simulink model "Hinf_sim"  (R2020a)
settings: Solver=VariableStepAuto  StartTime=0.0  StopTime=T  MaxStep=dtmax  RelTol=1e-3
values from neighbouring files (symbols this model uses):
  b = b*b_error_scale    (= 131.4)    [Hinf_run.m]    (also in adaptive_control_run.m; passivity_fmod_run.m; passivity_velmod_run.m)
  C1 = balreal(K(1,2))    [Hinf_run.m]
  C2 = balreal(-inv(C1)*K(1,1))    [Hinf_run.m]
  input_type = 3    [Hinf_run.m]    (also in adaptive_control_run.m; passivity_fmod_run.m; passivity_velmod_run.m)
  k = k*k_error_scale    (= 11691)    [Hinf_run.m]    (also in adaptive_control_run.m; passivity_fmod_run.m; passivity_velmod_run.m)
  m = 500    [Hinf_run.m]    (also in adaptive_control_run.m; passivity_fmod_run.m; passivity_velmod_run.m)
  rampslope = 0.1    [Hinf_run.m]    (also in adaptive_control_run.m; passivity_fmod_run.m; passivity_velmod_run.m)
  sineamp = 0.1    [Hinf_run.m]    (also in adaptive_control_run.m; passivity_fmod_run.m; passivity_velmod_run.m)
  sinefreq = pi/2    (= 1.57079632679)    [Hinf_run.m]    (also in adaptive_control_run.m; passivity_fmod_run.m; passivity_velmod_run.m)
  taum = taum*taum_error_scale    (= 0.108)    [Hinf_run.m]    (also in adaptive_control_run.m; passivity_fmod_run.m; passivity_velmod_run.m)
settings Model: Creator=davidcarabis  LastModifiedBy=davidcarabis
settings DataIOCC: ReturnWorkspaceOutputs=off
settings DebuggingCC: ArithmeticOperatorsInVariantConditions=warning
settings SFSimCC: CustomCodeUndefinedFunction=UseInterfaceOnly

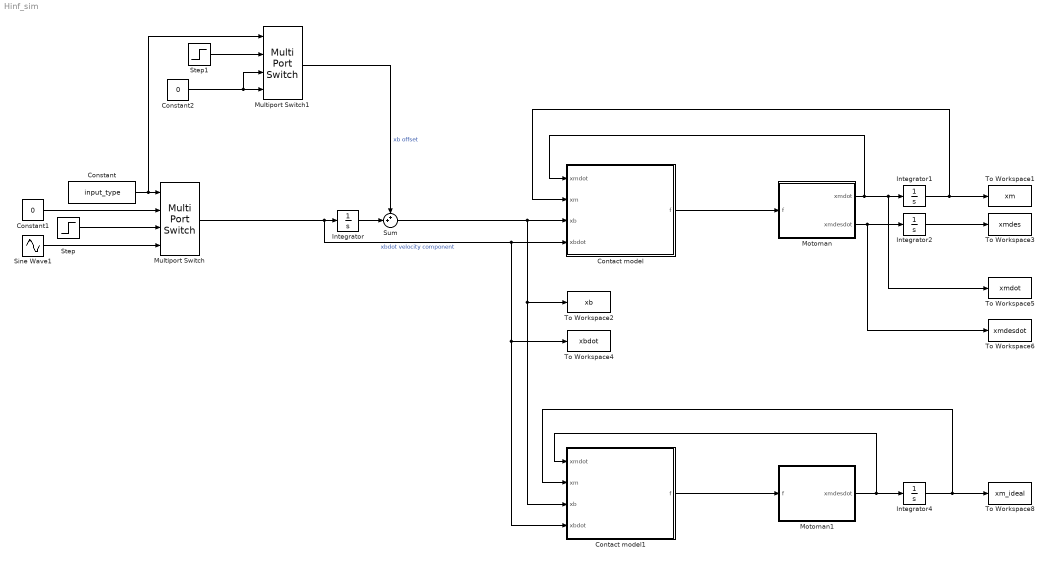
== system Hinf_sim ==
  Constant : Constant  Value=input_type
  Constant1 : Constant  Value=0
  Constant2 : Constant  Value=0
  Contact model : Subsystem
  Contact model1 : Subsystem
  Integrator{,1..2,4} (4 alike) : Integrator
  Motoman : Subsystem
  Motoman1 : Subsystem
  Multiport Switch : MultiPortSwitch
  Multiport Switch1 : MultiPortSwitch
  Sine Wave1 : Sin  Amplitude=sineamp*sinefreq  Frequency=sinefreq  Phase=pi/2  SampleTime=0
  Step : Step  Time=0  After=rampslope  SampleTime=0
  Step1 : Step  Time=0  After=rampslope  SampleTime=0
  Sum : Sum  Inputs=++|
  To Workspace1 : ToWorkspace  VariableName=xm  SampleTime=-1
  To Workspace2 : ToWorkspace  VariableName=xb
  To Workspace3 : ToWorkspace  VariableName=xmdes  SampleTime=-1
  To Workspace4 : ToWorkspace  VariableName=xbdot
  To Workspace5 : ToWorkspace  VariableName=xmdot  SampleTime=-1
  To Workspace6 : ToWorkspace  VariableName=xmdesdot  SampleTime=-1
  To Workspace8 : ToWorkspace  VariableName=xm_ideal  SampleTime=-1
  wires:
  Multiport Switch/1 -> Contact model1/4(xbdot), To Workspace4/1, Contact model/4(xbdot), Integrator/1  "xbdot velocity component"
  Constant/1 -> Multiport Switch1/1, Multiport Switch/1
  Step/1 -> Multiport Switch/3
  Sine Wave1/1 -> Multiport Switch/4
  Constant1/1 -> Multiport Switch/2
  Multiport Switch1/1 -> Sum/1  "xb offset"
  Integrator/1 -> Sum/2
  Constant2/1 -> Multiport Switch1/3, Multiport Switch1/4
  Step1/1 -> Multiport Switch1/2
  Motoman/1(xmdot) -> To Workspace5/1, Integrator1/1, Contact model/1(xmdot)
  Integrator1/1 -> Contact model/2(xm), To Workspace1/1
  Integrator2/1 -> To Workspace3/1
  Contact model/1(f) -> Motoman/1(f)
  Motoman/2(xmdesdot) -> To Workspace6/1, Integrator2/1
  Integrator4/1 -> Contact model1/2(xm), To Workspace8/1
  Contact model1/1(f) -> Motoman1/1(f)
  Motoman1/1(xmdesdot) -> Contact model1/1(xmdot), Integrator4/1
  Sum/1 -> Contact model1/3(xb), To Workspace2/1, Contact model/3(xb)

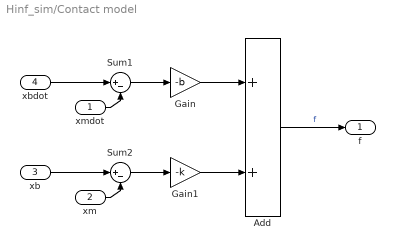
== system Hinf_sim/Contact model ==
  xmdot : Inport
  xm : Inport  Port=2
  xb : Inport  Port=3
  xbdot : Inport  Port=4
  Add : Sum
  Gain : Gain  Gain=-b
  Gain1 : Gain  Gain=-k
  Sum1 : Sum  Inputs=|+-
  Sum2 : Sum  Inputs=|+-
  f : Outport  VectorParamsAs1DForOutWhenUnconnected=off
  wires:
  xmdot/1 -> Sum1/2
  Add/1 -> f/1  "f"
  Sum2/1 -> Gain1/1
  xb/1 -> Sum2/1
  Gain1/1 -> Add/2
  Sum1/1 -> Gain/1
  xbdot/1 -> Sum1/1
  Gain/1 -> Add/1
  xm/1 -> Sum2/2

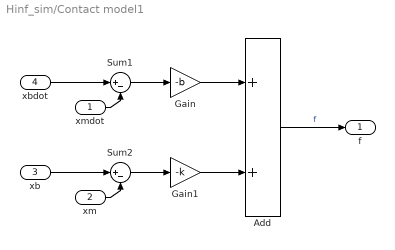
== system Hinf_sim/Contact model1 ==
  xmdot : Inport
  xm : Inport  Port=2
  xb : Inport  Port=3
  xbdot : Inport  Port=4
  Add : Sum
  Gain : Gain  Gain=-b
  Gain1 : Gain  Gain=-k
  Sum1 : Sum  Inputs=|+-
  Sum2 : Sum  Inputs=|+-
  f : Outport  VectorParamsAs1DForOutWhenUnconnected=off
  wires:
  xmdot/1 -> Sum1/2
  Add/1 -> f/1  "f"
  Sum2/1 -> Gain1/1
  xb/1 -> Sum2/1
  Gain1/1 -> Add/2
  Sum1/1 -> Gain/1
  xbdot/1 -> Sum1/1
  Gain/1 -> Add/1
  xm/1 -> Sum2/2

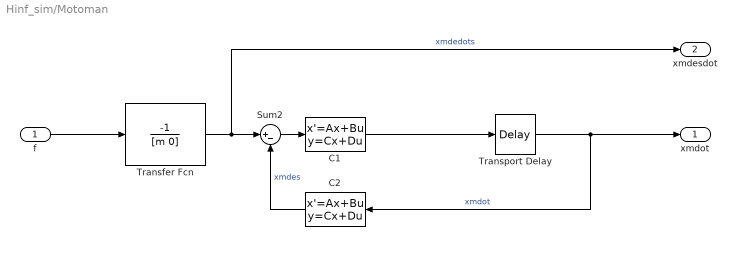
== system Hinf_sim/Motoman ==
  f : Inport
  C1 : StateSpace  A=C1.A  B=C1.B  C=C1.C  D=C1.D  InitialCondition=0
  C2 : StateSpace  A=C2.A  B=C2.B  C=C2.C  D=C2.D  InitialCondition=0
  Sum2 : Sum  Inputs=|+-
  Transfer Fcn : TransferFcn  Numerator=[-1]  Denominator=[m 0]
  Transport Delay : TransportDelay  DelayTime=taum
  xmdot : Outport  VectorParamsAs1DForOutWhenUnconnected=off
  xmdesdot : Outport  Port=2  VectorParamsAs1DForOutWhenUnconnected=off
  wires:
  f/1 -> Transfer Fcn/1
  Transport Delay/1 -> C2/1, xmdot/1  "xmdot"
  Transfer Fcn/1 -> xmdesdot/1, Sum2/1  "xmdedots"
  Sum2/1 -> C1/1
  C2/1 -> Sum2/2  "xmdes"
  C1/1 -> Transport Delay/1

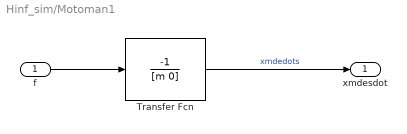
== system Hinf_sim/Motoman1 ==
  f : Inport
  Transfer Fcn : TransferFcn  Numerator=[-1]  Denominator=[m 0]
  xmdesdot : Outport  VectorParamsAs1DForOutWhenUnconnected=off
  wires:
  f/1 -> Transfer Fcn/1
  Transfer Fcn/1 -> xmdesdot/1  "xmdedots"
